simulink model "A2Model"  (R2015b)
settings: Solver=VariableStepAuto  StartTime=0.0  StopTime=inf  RelTol=1e-3
model workspace (MAT data in the model file):
  GPSLL = Simulink.Parameter
  GPSLL.Value = [47.255 11.345]
  GPSLL.DataType = 'auto'
  GPSLL.Units = 'auto'
  Inertia = Simulink.Parameter
  Inertia.Value = [0.035  0  0; 0  0.035  0; 0  0  0.011]
  Inertia.DataType = 'auto'
  Inertia.Units = 'auto'
  Mass = Simulink.Parameter
  Mass.Value = 1.5
  Mass.DataType = 'auto'
  Mass.Units = 'auto'
undefined symbols (not defined in the file): Earth, FilterK, PitchKd, PitchKi, PitchKp, PitchMax, Receive, RollKd, RollKi, RollKp, RollMax, Send, sigbuilder_block, Ts, WGS84
libraries: simulink x15, aerolibfltsims x5, simulink_extras x4, aerolibanimutils x2, aerolibtransform2 x2, aerolibconvert2 x2, aerolib6dof2 x1, aerolibatmos2 x1
settings Model: Creator=Ivan  LastModifiedBy=Ivan
settings OptimizationCC: DefaultParameterBehavior=Inlined  UseFloatMulNetSlope=on  InlineInvariantSignals=on  PassReuseOutputArgsAs=Individual arguments  ZeroExternalMemoryAtStartup=off  ZeroInternalMemoryAtStartup=off  NoFixptDivByZeroProtection=on  EfficientFloat2IntCast=on  OptimizeModelRefInitCode=on  LifeSpan=1
settings DebuggingCC: ParameterPrecisionLossMsg=none
settings HardwareCC: ProdBitPerPointer=32  ProdLargestAtomicInteger=Long  ProdLargestAtomicFloat=Double  ProdWordSize=32  ProdHWDeviceType=ARM Compatible->ARM Cortex
settings RTWCC: SystemTargetFile=ert.tlc  TemplateMakefile=ert_default_tmf  Description=Embedded Coder  GenerateReport=on  IncludeHyperlinkInReport=on  LaunchReport=on  TargetLang=C++  GenerateTraceInfo=on  GenerateTraceReport=on  GenerateTraceReportSl=on  GenerateTraceReportSf=on  GenerateTraceReportEml=on
settings CodeAppCC: ForceParamTrailComments=on  IgnoreCustomStorageClasses=off  SimulinkDataObjDesc=on  CustomSymbolStrGlobalVar=rt$N$M  CustomSymbolStrType=$N$M  CustomSymbolStrFcn=$N$M$F  CustomSymbolStrMacro=$N$M  InsertBlockDesc=on
settings ERTTargetCC: GenerateSampleERTMain=on  IncludeMdlTerminateFcn=off  CombineSignalStateStructs=on  MultiInstanceERTCode=on  CodeInterfacePackaging=C++ class  SupportNonFinite=off  SupportComplex=off  InlinedParameterPlacement=NonHierarchical  RootIOFormat=Structure reference  ERTCustomFileTemplate=example_file_process.tlc  ERTFilePackagingFormat=CompactWithDataFile

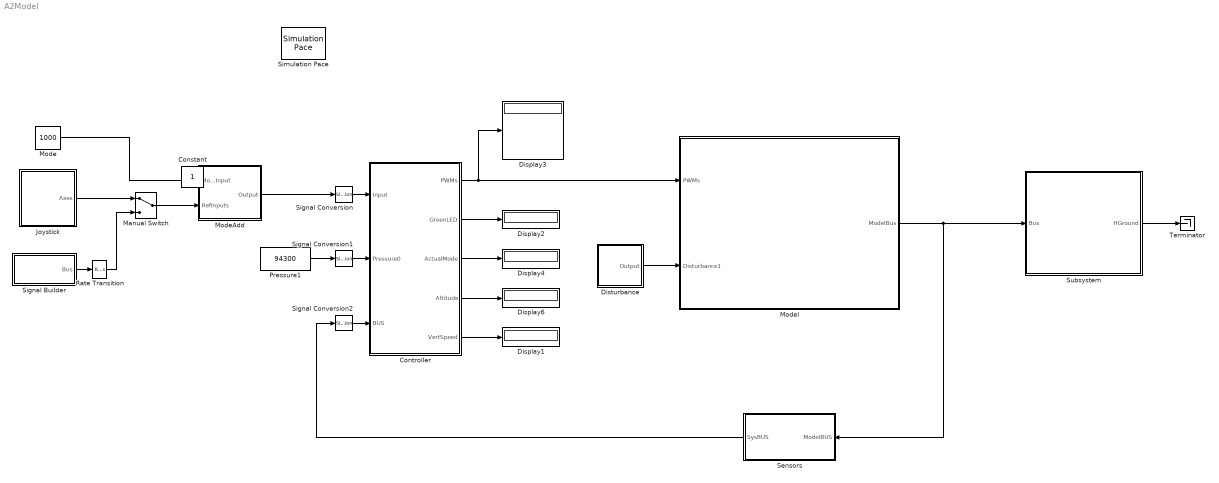
== system A2Model ==
  Controller : Subsystem  TreatAsAtomicUnit=on  SystemSampleTime=Ts
  Display{1..4,6} (5 alike) : Display
  Disturbance : Subsystem
  Joystick : Subsystem
  Manual Switch : ManualSwitch
  Mode : Constant  Value=1000  OutDataTypeStr=uint32  SampleTime=Ts
  ModeAdd : Subsystem
  Model : Subsystem
  Pressure1 : Constant  Value=94300  OutDataTypeStr=single  SampleTime=Ts
  Rate Transition : RateTransition  OutPortSampleTime=Ts
  Sensors : Subsystem
  Signal Conversion : SignalConversion
  Signal Conversion1 : SignalConversion
  Signal Conversion2 : SignalConversion
  Signal Builder : Subsystem  Tag=STV Subsys  LoadFcn=sigbuilder_block('load');  StartFcn=sigbuilder_block('start');  StopFcn=sigbuilder_block('stop');  ClipboardFcn=sigbuilder_block('clipboard');  mask(Sigbuilder block){}
      mask help: Simulink:masks:SigbuilderBlock_MD
      mask init:
      | if ~strcmp(get_param(bdroot(gcbh),'SimulationStatus'),'stopped') tuvar = sigbuilder_block('maskInit'); end
      settings: CopyFcn=sigbuilder_block('copy');  DeleteFcn=sigbuilder_block('delete');  ModelCloseFcn=sigbuilder_block('modelClose');  PreSaveFcn=sigbuilder_block('preSave');  PauseFcn=sigbuilder_block('pause');  ContinueFcn=sigbuilder_block('continue');  NameChangeFcn=sigbuilder_block('namechange');  OpenFcn=sigbuilder_block('open',[489.5 178 830 726.5 ]);  CloseFcn=sigbuilder_block('close');
      mask Display: plot(0, 0, 100, 100,[2, 2, 32, 32, 2], [68, 8, 8, 68, 68],[32, 2], [38, 38], [32, 19, 2],[53, 60, 44], [32, 17, 17, 2],[16, 16, 31, 31]);txt = getActiveGroup(gcbh);text(2, 100, txt,'verticalAlignment', 'top');
  Simulation Pace : aerolibanimutils/Simulation Pace  SimulationPace=1  SleepMode=MATLAB Thread  OutputPaceError=off  SampleTime=Ts
  Subsystem : Subsystem
  Terminator : Terminator
  Constant : Constant  IOType=siggen
  wires:
  Mode/1 -> ModeAdd/1(ModeInput)
  Joystick/1(Axes) -> Manual Switch/1
  Manual Switch/1 -> ModeAdd/2(RefInputs)
  Signal Builder/1(Bus) -> Rate Transition/1
  Rate Transition/1 -> Manual Switch/2
  Disturbance/1(Output) -> Model/2(Disturbance1)
  Controller/1(PWMs) -> Model/1(PWMs), Display3/1
  Model/1(ModelBus) -> Subsystem/1(Bus), Sensors/1(ModelBUS)
  Sensors/1(SysBUS) -> Signal Conversion2/1
  Controller/4(Altitude) -> Display6/1
  Controller/5(VertSpeed) -> Display1/1
  Controller/2(GreenLED) -> Display2/1
  Pressure1/1 -> Signal Conversion1/1
  Controller/3(ActualMode) -> Display4/1
  Signal Conversion/1 -> Controller/1(Input)
  Signal Conversion1/1 -> Controller/2(Pressure0)
  Signal Conversion2/1 -> Controller/3(BUS)
  Subsystem/1(HGround) -> Terminator/1
  ModeAdd/1(Output) -> Signal Conversion/1

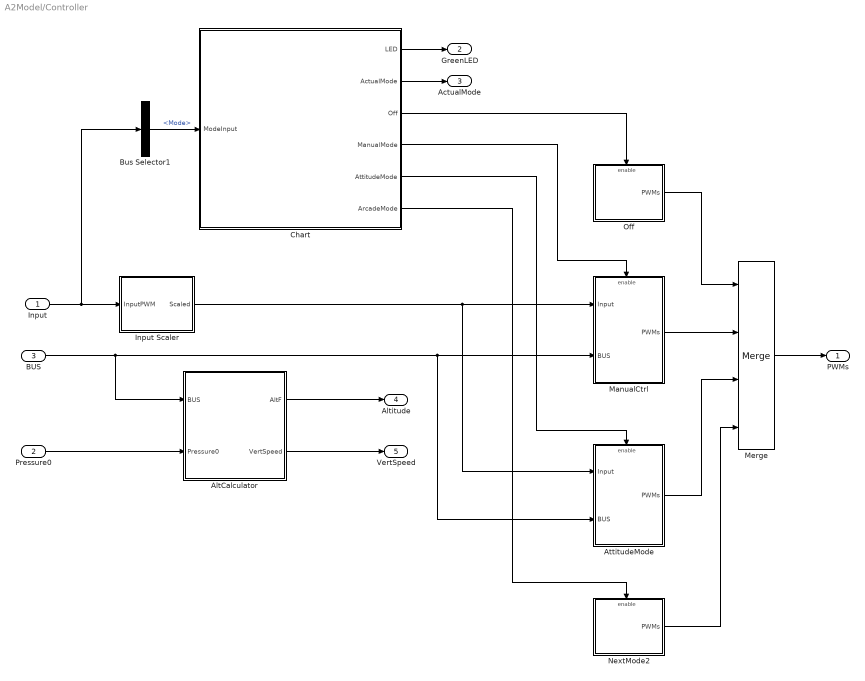
== system A2Model/Controller ==
  Input : Inport
  Pressure0 : Inport  Port=2
  BUS : Inport  Port=3
  AltCalculator : Subsystem
  AttitudeMode : Subsystem
  Bus Selector1 : BusSelector  OutputSignals=Mode
  Chart : Stateflow chart  TreatAsAtomicUnit=on
  Input Scaler : Subsystem
  ManualCtrl : Subsystem
  Merge : Merge  Inputs=4
  NextMode2 : Subsystem
  Off : Subsystem
  PWMs : Outport
  GreenLED : Outport  Port=2
  ActualMode : Outport  Port=3
  Altitude : Outport  Port=4
  VertSpeed : Outport  Port=5
  wires:
  Input/1 -> Bus Selector1/1, Input Scaler/1(InputPWM)
  BUS/1 -> ManualCtrl/2(BUS), AttitudeMode/2(BUS), AltCalculator/1(BUS)
  AltCalculator/2(VertSpeed) -> VertSpeed/1
  AltCalculator/1(AltF) -> Altitude/1
  Pressure0/1 -> AltCalculator/2(Pressure0)
  Input Scaler/1(Scaled) -> AttitudeMode/1(Input), ManualCtrl/1(Input)
  Chart/1(LED) -> GreenLED/1
  Bus Selector1/1 -> Chart/1(ModeInput)  "<Mode>"
  ManualCtrl/1(PWMs) -> Merge/2
  Off/1(PWMs) -> Merge/1
  Merge/1 -> PWMs/1
  Chart/2(ActualMode) -> ActualMode/1
  Chart/4(" ManualMode") -> ManualCtrl/Enable
  AttitudeMode/1(PWMs) -> Merge/3
  Chart/3(" Off") -> Off/Enable
  Chart/5(" AttitudeMode") -> AttitudeMode/Enable
  Chart/6(" ArcadeMode") -> NextMode2/Enable
  NextMode2/1(PWMs) -> Merge/4

== system A2Model/Disturbance ==
  Mode3 : Constant  Value=[0 0 0]  OutDataTypeStr=Inherit: Inherit via back propagation  SampleTime=Ts
  Mux : Mux  Inputs=2
  Step : Step  Time=10  Before=[0 0 0]  After=[0 0 0]  SampleTime=0
  Output : Outport
  wires:
  Step/1 -> Mux/1  "F[N]"
  Mux/1 -> Output/1
  Mode3/1 -> Mux/2  "Torque"

== system A2Model/Joystick ==
  Bus Creator : BusCreator  Inputs=4
  Joy Scaler : Subsystem
  Joystick : Subsystem
  Terminator{,1..3} (4 alike) : Terminator
  Axes : Outport
  wires:
  Joystick/1(Roll) -> Bus Creator/1  "Roll"
  Joystick/2(Pitch) -> Bus Creator/2  "Pitch"
  Joystick/3(Yaw) -> Bus Creator/3  "Yaw"
  Joystick/4(Throttle) -> Bus Creator/4  "Throttle"
  Bus Creator/1 -> Joy Scaler/1(Joystick)
  Joystick/7(B3) -> Terminator3/1
  Joystick/6(B2) -> Terminator1/1
  Joystick/5(B1) -> Terminator/1
  Joystick/8(B4) -> Terminator2/1
  Joy Scaler/1(Scaled) -> Axes/1

== system A2Model/ModeAdd ==
  ModeInput : Inport
  RefInputs : Inport  Port=2
  Bus Creator : BusCreator  Inputs=5
  Bus Selector2 : BusSelector  OutputSignals=Thr,Aileron,Elevator,Rudder
  Data Type Conversion{,1..3} (4 alike) : DataTypeConversion  OutDataTypeStr=single
  Output : Outport
  wires:
  Bus Selector2/1 -> Data Type Conversion/1  "<Thr>"
  Bus Selector2/2 -> Data Type Conversion1/1  "<Aileron>"
  RefInputs/1 -> Bus Selector2/1
  Bus Selector2/3 -> Data Type Conversion2/1  "<Elevator>"
  Bus Selector2/4 -> Data Type Conversion3/1  "<Rudder>"
  Bus Creator/1 -> Output/1
  ModeInput/1 -> Bus Creator/1  "Mode"
  Data Type Conversion/1 -> Bus Creator/2  "Thr"
  Data Type Conversion1/1 -> Bus Creator/3  "Aileron"
  Data Type Conversion2/1 -> Bus Creator/4  "Elevator"
  Data Type Conversion3/1 -> Bus Creator/5  "Rudder"

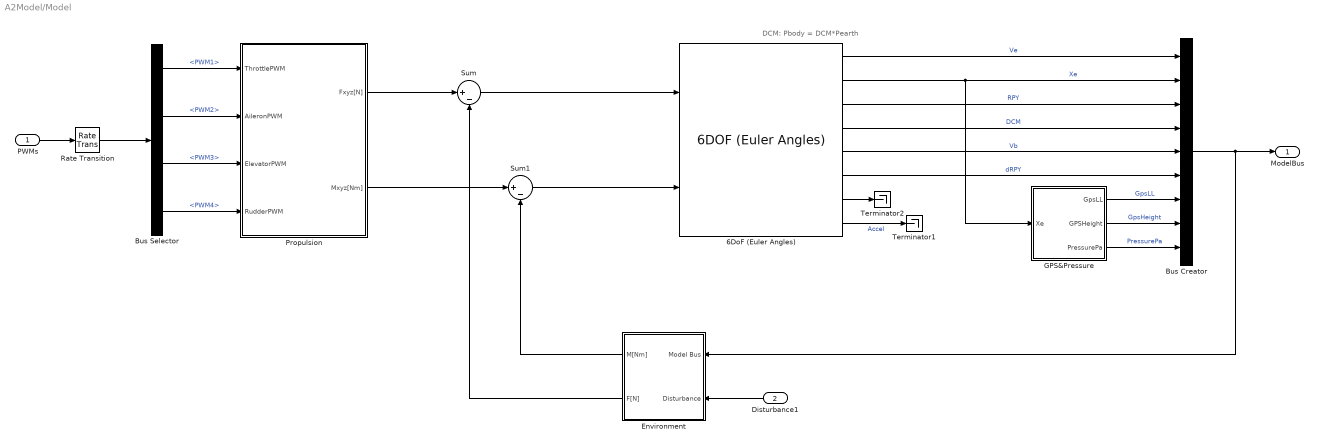
== system A2Model/Model ==
  note: DCM:
      | Pbody = DCM*Pearth
  PWMs : Inport
  Disturbance1 : Inport  Port=2
  6DoF (Euler Angles) : aerolib6dof2/6DOF (Euler Angles)  units=Metric (MKS)  mtype=Fixed  rep=Euler Angles  xme_0=[0 0 -600]  Vm_0=[0 0 0]  eul_0=[0 0 0]  pm_0=[0 0 0]  mass_0=Mass  mass_e=0.5  mass_f=2.0  inertia=Inertia  inertia_e=eye(3)  inertia_f=2*eye(3)  k_quat=1.0  vre_flag=on
  Bus Creator : BusCreator  Inputs=9
  Bus Selector : BusSelector  OutputSignals=PWM1,PWM2,PWM3,PWM4
  Environment : Subsystem
  GPS&Pressure : Subsystem
  Propulsion : Subsystem
  Rate Transition : RateTransition
  Sum : Sum  Inputs=|+-
  Sum1 : Sum  Inputs=|+-
  Terminator1 : Terminator
  Terminator2 : Terminator
  ModelBus : Outport
  wires:
  6DoF (Euler Angles)/1 -> Bus Creator/1  "Ve"
  6DoF (Euler Angles)/2 -> GPS&Pressure/1(Xe), Bus Creator/2  "Xe"
  6DoF (Euler Angles)/3 -> Bus Creator/3  "RPY"
  6DoF (Euler Angles)/4 -> Bus Creator/4  "DCM"
  Propulsion/2(Mxyz[Nm]) -> Sum1/1
  Propulsion/1(Fxyz[N]) -> Sum/1
  6DoF (Euler Angles)/7 -> Terminator2/1
  PWMs/1 -> Rate Transition/1
  Bus Selector/1 -> Propulsion/1(ThrottlePWM)  "<PWM1>"
  Bus Selector/2 -> Propulsion/2(AileronPWM)  "<PWM2>"
  Bus Selector/3 -> Propulsion/3(ElevatorPWM)  "<PWM3>"
  Bus Selector/4 -> Propulsion/4(RudderPWM)  "<PWM4>"
  Sum/1 -> 6DoF (Euler Angles)/1
  6DoF (Euler Angles)/5 -> Bus Creator/5  "Vb"
  6DoF (Euler Angles)/6 -> Bus Creator/6  "dRPY"
  Rate Transition/1 -> Bus Selector/1
  6DoF (Euler Angles)/8 -> Terminator1/1  "Accel"
  GPS&Pressure/1(GpsLL) -> Bus Creator/7  "GpsLL"
  GPS&Pressure/2(GPSHeight) -> Bus Creator/8  "GpsHeight"
  GPS&Pressure/3(PressurePa) -> Bus Creator/9  "PressurePa"
  Bus Creator/1 -> Environment/1(Model Bus), ModelBus/1
  Disturbance1/1 -> Environment/2(Disturbance)
  Sum1/1 -> 6DoF (Euler Angles)/2
  Environment/1(M[Nm]) -> Sum1/2
  Environment/2(F[N]) -> Sum/2

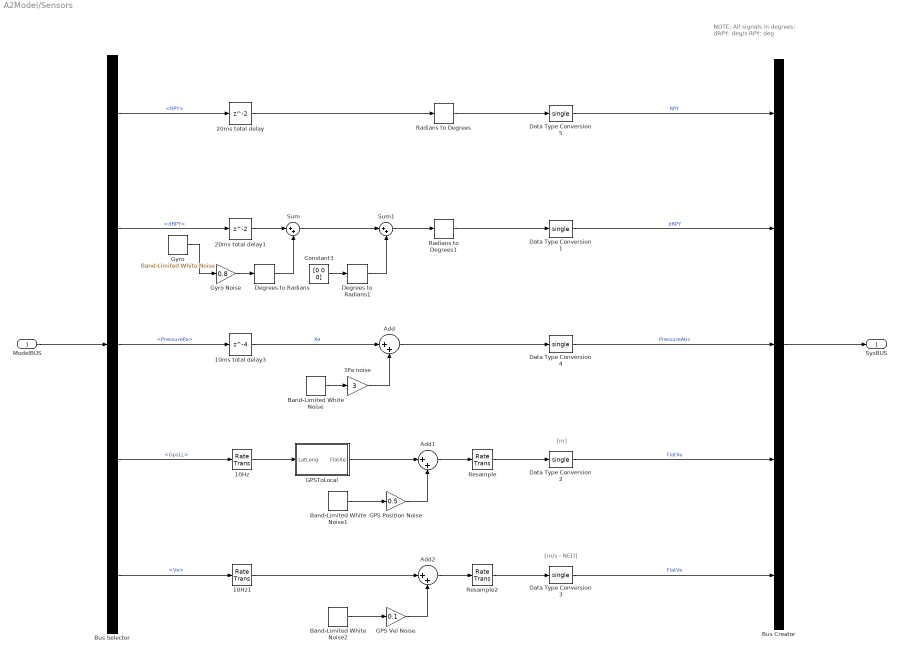
== system A2Model/Sensors ==
  note: [m/s - NED]
  note: [m]
  note: NOTE: All signals in degrees:
      | dRPY: deg/s
      | RPY: deg
  ModelBUS : Inport
  10Hz : RateTransition  OutPortSampleTime=1/10
  10Hz1 : RateTransition  OutPortSampleTime=1/10
  10ms total delay3 : Delay  DelayLength=4  SampleTime=Ts
  20ms total delay : Delay  SampleTime=Ts
  20ms total delay1 : Delay  SampleTime=Ts
  3Pa noise : Gain  Gain=3
  Add : Sum  Inputs=|++
  Add1 : Sum  Inputs=|++
  Add2 : Sum  Inputs=|++
  Band-Limited White Noise : simulink/Sources/Band-Limited White Noise  Cov=[1]*Ts  Ts=Ts  seed=[23341]
  Band-Limited White Noise1 : simulink/Sources/Band-Limited White Noise  Cov=[1]*Ts  Ts=Ts  seed=[23341]
  Band-Limited White Noise2 : simulink/Sources/Band-Limited White Noise  Cov=[1]*Ts  Ts=Ts  seed=[23341]
  Bus Creator : BusCreator  Inputs=5
  Bus Selector : BusSelector  OutputSignals=RPY,dRPY,PressurePa,GpsLL,Ve
  Constant3 : Constant  Value=[0 0 0]  OutDataTypeStr=single
  Data Type Conversion{1..5} (5 alike) : DataTypeConversion  OutDataTypeStr=single
  Degrees to Radians : simulink_extras/Transformations/Degrees to Radians
  Degrees to Radians1 : simulink_extras/Transformations/Degrees to Radians
  GPS Position Noise : Gain  Gain=0.5
  GPS Vel Noise : Gain  Gain=0.1
  GPSToLocal : Subsystem
  Gyro : simulink/Sources/Band-Limited White Noise  Cov=[1]*Ts  Ts=Ts  seed=[23341]
  Gyro Noise : Gain  Gain=0.8
  Radians to Degrees : simulink_extras/Transformations/Radians to Degrees
  Radians to Degrees1 : simulink_extras/Transformations/Radians to Degrees
  Resample : RateTransition  OutPortSampleTime=Ts
  Resample2 : RateTransition  OutPortSampleTime=Ts
  Sum : Sum  Inputs=|++
  Sum1 : Sum  Inputs=|++
  SysBUS : Outport
  wires:
  ModelBUS/1 -> Bus Selector/1
  Bus Selector/1 -> 20ms total delay/1  "<RPY>"
  Bus Creator/1 -> SysBUS/1
  Bus Selector/2 -> 20ms total delay1/1  "<dRPY>"
  20ms total delay/1 -> Radians to Degrees/1
  20ms total delay1/1 -> Sum/1
  Gyro/1 -> Gyro Noise/1
  Data Type Conversion5/1 -> Bus Creator/1  "RPY"
  Data Type Conversion1/1 -> Bus Creator/2  "dRPY"
  Degrees to Radians/1 -> Sum/2
  Radians to Degrees/1 -> Data Type Conversion5/1
  Radians to Degrees1/1 -> Data Type Conversion1/1
  Sum/1 -> Sum1/1
  Sum1/1 -> Radians to Degrees1/1
  Constant3/1 -> Degrees to Radians1/1
  Degrees to Radians1/1 -> Sum1/2
  Data Type Conversion3/1 -> Bus Creator/5  "FlatVe"
  Data Type Conversion2/1 -> Bus Creator/4  "FlatXe"
  3Pa noise/1 -> Add/2
  Band-Limited White Noise/1 -> 3Pa noise/1
  Add/1 -> Data Type Conversion4/1
  10ms total delay3/1 -> Add/1  "Xe"
  Bus Selector/3 -> 10ms total delay3/1  "<PressurePa>"
  Data Type Conversion4/1 -> Bus Creator/3  "PressureAbs"
  Bus Selector/4 -> 10Hz/1  "<GpsLL>"
  Bus Selector/5 -> 10Hz1/1  "<Ve>"
  10Hz/1 -> GPSToLocal/1(LatLong)
  Resample/1 -> Data Type Conversion2/1
  Resample2/1 -> Data Type Conversion3/1
  GPS Position Noise/1 -> Add1/2
  Band-Limited White Noise1/1 -> GPS Position Noise/1
  GPSToLocal/1(FlatXe) -> Add1/1
  Add1/1 -> Resample/1
  GPS Vel Noise/1 -> Add2/2
  Band-Limited White Noise2/1 -> GPS Vel Noise/1
  10Hz1/1 -> Add2/1
  Add2/1 -> Resample2/1
  Gyro Noise/1 -> Degrees to Radians/1

== system A2Model/Signal Builder ==
  Bus Creator : BusCreator  Tag=Bus Creator  Inputs=4
  FromWs : FromWorkspace  Tag=STV FromWs  VariableName=tuvar  SampleTime=0
      SigBuilderData=|
      | common.afterFinalStr = 'Extrapolate'
      | common.sampleTime = 0
      | dataSet.timeRange = [0 20]
      | dataSet.name = 'Group 1'
      | sbobj.Groups.Name = 'Group 1'
      | sbobj.Groups.Signals(1).Name = 'Thr'
      | sbobj.Groups.Signals(1).XData = [0 20]
      | sbobj.Groups.Signals(1).YData = [1300 1300]
      | sbobj.Groups.Signals(2).Name = 'Aileron'
      | sbobj.Groups.Signals(2).XData = [0 20]
      | sbobj.Groups.Signals(2).YData = [1024 1024]
      | sbobj.Groups.Signals(3).Name = 'Elevator'
      | sbobj.Groups.Signals(3).XData = [0 20]
      | sbobj.Groups.Signals(3).YData = [1024 1024]
      | sbobj.Groups.Signals(4).Name = 'Rudder'
      | sbobj.Groups.Signals(4).XData = [0 20]
      | sbobj.Groups.Signals(4).YData = [1024 1024]
      | sbobj.Groups.TimeRange = [0 20]
  Subsystem : Subsystem
  Bus : Outport
  wires:
  FromWs/1 -> Subsystem/1(In1)
  Subsystem/1(Thr) -> Bus Creator/1  "Thr"
  Subsystem/2(Aileron) -> Bus Creator/2  "Aileron"
  Subsystem/3(Elevator) -> Bus Creator/3  "Elevator"
  Subsystem/4(Rudder) -> Bus Creator/4  "Rudder"
  Bus Creator/1 -> Bus/1

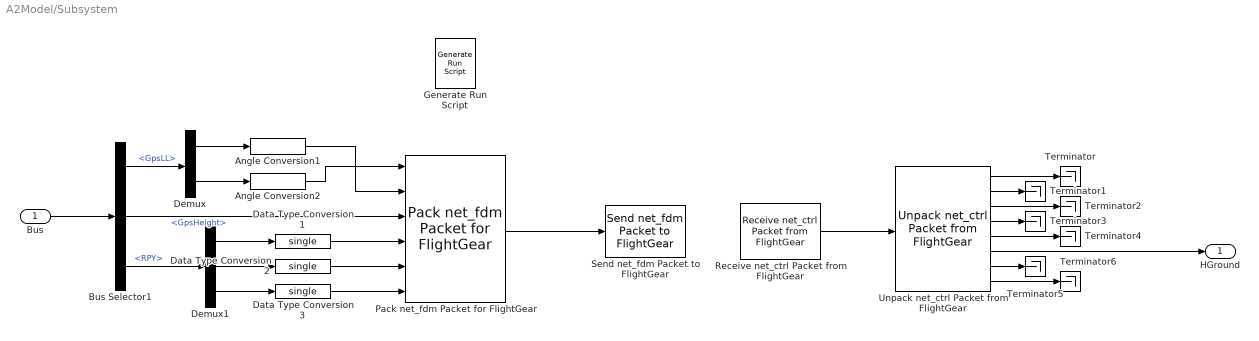
== system A2Model/Subsystem ==
  Bus : Inport
  Angle Conversion1 : aerolibconvert2/Angle Conversion  IU=deg  OU=rad
  Angle Conversion2 : aerolibconvert2/Angle Conversion  IU=deg  OU=rad
  Bus Selector1 : BusSelector  OutputSignals=GpsLL,GpsHeight,RPY
  Data Type Conversion1 : DataTypeConversion  OutDataTypeStr=single
  Data Type Conversion2 : DataTypeConversion  OutDataTypeStr=single
  Data Type Conversion3 : DataTypeConversion  OutDataTypeStr=single
  Demux : Demux  Outputs=2
  Demux1 : Demux  Outputs=3
  Generate Run Script : aerolibfltsims/Generate Run Script  OutputFileName=runfg.bat  FlightGearBaseDirectory=C:\Program Files\FlightGear 3.4.0  GeometryModelName=Kiki  DestinationPort=5502  OriginAddress=127.0.0.1  OriginPort=5505  LocalAddress=127.0.0.1  AirportId=LDZA  RunwayId=16  InitialAltitude=5000  InitialHeading=0  OffsetDistance=0  OffsetAzimuth=0  GenerateFile=off  Architecture=Win64  dataFlow=Send-Receive
  Pack net_fdm Packet for FlightGear : aerolibfltsims/Pack net_fdm Packet for FlightGear  FlightGearVersion=v3.4  ShowPositionAttitudeInputs=on  ShowVelocityAccelerationInputs=off  ShowControlSurfacePositionInputs=off  ShowEngineFuelInputs=off  ShowLandingGearInputs=off  ShowEnvironmentInputs=off  SampleTime=1/30
  Receive net_ctrl Packet from FlightGear : aerolibfltsims/Receive net_ctrl Packet from FlightGear  FlightGearVersion=v3.4  ReceiveAddress=127.0.0.1  ReceivePort=5505  ReceiveWidth=744  varLen=off  SampleTime=1/30  packetFlag=off
      settings: AttributesFormatString=Version Selected:\n%<FlightGearVersion>
  Send net_fdm Packet to FlightGear : aerolibfltsims/Send net_fdm Packet to FlightGear  DestinationIpAddress=127.0.0.1  DestinationPort=5502  LocalIpPort=-1  varLen=off  SampleTime=1/30
  Terminator{,1..6} (7 alike) : Terminator
  Unpack net_ctrl Packet from FlightGear : aerolibfltsims/Unpack net_ctrl Packet from FlightGear  FlightGearVersion=v3.4  ShowControlSurfacePositionOutputs=off  ShowEngineFuelOutputs=off  ShowLandingGearOutputs=off  ShowAvionicOutputs=off  ShowEnvironmentOutputs=on  SampleTime=1/30
      settings: AttributesFormatString=Version Selected: %<FlightGearVersion>
  HGround : Outport
  wires:
  Pack net_fdm Packet for FlightGear/1 -> Send net_fdm Packet to FlightGear/1
  Bus/1 -> Bus Selector1/1
  Bus Selector1/1 -> Demux/1  "<GpsLL>"
  Demux/1 -> Angle Conversion1/1
  Demux/2 -> Angle Conversion2/1
  Bus Selector1/2 -> Pack net_fdm Packet for FlightGear/3  "<GpsHeight>"
  Demux1/1 -> Data Type Conversion1/1
  Demux1/2 -> Data Type Conversion2/1
  Demux1/3 -> Data Type Conversion3/1
  Data Type Conversion1/1 -> Pack net_fdm Packet for FlightGear/4
  Data Type Conversion2/1 -> Pack net_fdm Packet for FlightGear/5
  Data Type Conversion3/1 -> Pack net_fdm Packet for FlightGear/6
  Bus Selector1/3 -> Demux1/1  "<RPY>"
  Receive net_ctrl Packet from FlightGear/1 -> Unpack net_ctrl Packet from FlightGear/1
  Unpack net_ctrl Packet from FlightGear/6 -> HGround/1
  Angle Conversion1/1 -> Pack net_fdm Packet for FlightGear/2
  Angle Conversion2/1 -> Pack net_fdm Packet for FlightGear/1
  Unpack net_ctrl Packet from FlightGear/1 -> Terminator/1
  Unpack net_ctrl Packet from FlightGear/2 -> Terminator1/1
  Unpack net_ctrl Packet from FlightGear/3 -> Terminator2/1
  Unpack net_ctrl Packet from FlightGear/4 -> Terminator3/1
  Unpack net_ctrl Packet from FlightGear/5 -> Terminator4/1
  Unpack net_ctrl Packet from FlightGear/7 -> Terminator5/1
  Unpack net_ctrl Packet from FlightGear/8 -> Terminator6/1

== system A2Model/Controller/AltCalculator ==
  BUS : Inport
  Pressure0 : Inport  Port=2
  Bus Selector1 : BusSelector  OutputSignals=PressureAbs
  Delay : Delay  DelayLength=100
  Discrete FIR Filter : DiscreteFir  Coefficients=FilterK
  Gain : Gain  Gain=1/(100*Ts)
  MATLAB Function : MATLAB Function  TreatAsAtomicUnit=on
  Sum : Sum  Inputs=|+-
  AltF : Outport
  VertSpeed : Outport  Port=2
  wires:
  BUS/1 -> Bus Selector1/1
  Bus Selector1/1 -> MATLAB Function/1(pressure)  "<PressureAbs>"
  MATLAB Function/1(alt) -> Discrete FIR Filter/1
  Sum/1 -> Gain/1
  Discrete FIR Filter/1 -> Delay/1, Sum/1, AltF/1
  Delay/1 -> Sum/2
  Gain/1 -> VertSpeed/1
  Pressure0/1 -> MATLAB Function/2(pressure0)

== system A2Model/Controller/AttitudeMode ==
  Input : Inport  OutDataTypeStr=single
  BUS : Inport  Port=2  OutDataTypeStr=single
  Enable : EnablePort  StatesWhenEnabling=reset
  Bus Selector1 : BusSelector  OutputSignals=Thr,Aileron,Elevator,Rudder
  Gain : Gain
  Gain3 : Gain
  Mapper : Subsystem
  PitchController : Subsystem
  RollController : Subsystem
  PWMs : Outport
  wires:
  Mapper/1(PwmOut) -> PWMs/1
  Gain/1 -> Mapper/1(Thr)
  Gain3/1 -> Mapper/4(Rudder)
  PitchController/1(PitchOut) -> Mapper/3(Elevator)
  Bus Selector1/4 -> Gain3/1  "<Rudder>"
  Input/1 -> Bus Selector1/1
  Bus Selector1/1 -> Gain/1  "<Thr>"
  Bus Selector1/3 -> PitchController/2(PitchRef)  "<Elevator>"
  BUS/1 -> PitchController/1(Bus), RollController/1(Bus)
  Bus Selector1/2 -> RollController/2(RollRef)  "<Aileron>"
  RollController/1(RollOut) -> Mapper/2(Aileron)

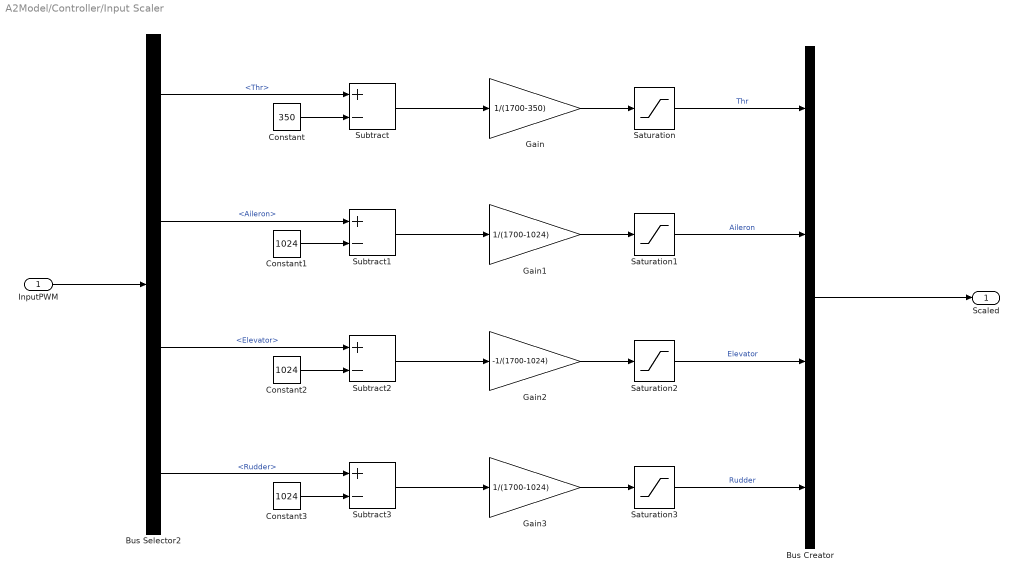
== system A2Model/Controller/Input Scaler ==
  InputPWM : Inport
  Bus Creator : BusCreator  Inputs=4
  Bus Selector2 : BusSelector  OutputSignals=Thr,Aileron,Elevator,Rudder
  Constant : Constant  Value=350  OutDataTypeStr=single
  Constant1 : Constant  Value=1024  OutDataTypeStr=single
  Constant2 : Constant  Value=1024  OutDataTypeStr=single
  Constant3 : Constant  Value=1024  OutDataTypeStr=single
  Gain : Gain  Gain=1/(1700-350)
  Gain1 : Gain  Gain=1/(1700-1024)
  Gain2 : Gain  Gain=-1/(1700-1024)
  Gain3 : Gain  Gain=1/(1700-1024)
  Saturation : Saturate  UpperLimit=1  LowerLimit=0
  Saturation1 : Saturate  UpperLimit=1  LowerLimit=-1
  Saturation2 : Saturate  UpperLimit=1  LowerLimit=-1
  Saturation3 : Saturate  UpperLimit=1  LowerLimit=-1
  Subtract{,1..3} (4 alike) : Sum  Inputs=+-
  Scaled : Outport
  wires:
  Bus Creator/1 -> Scaled/1
  InputPWM/1 -> Bus Selector2/1
  Bus Selector2/1 -> Subtract/1  "<Thr>"
  Constant/1 -> Subtract/2
  Subtract/1 -> Gain/1
  Gain/1 -> Saturation/1
  Saturation/1 -> Bus Creator/1  "Thr"
  Bus Selector2/2 -> Subtract1/1  "<Aileron>"
  Constant1/1 -> Subtract1/2
  Subtract1/1 -> Gain1/1
  Gain1/1 -> Saturation1/1
  Saturation1/1 -> Bus Creator/2  "Aileron"
  Bus Selector2/3 -> Subtract2/1  "<Elevator>"
  Constant2/1 -> Subtract2/2
  Subtract2/1 -> Gain2/1
  Gain2/1 -> Saturation2/1
  Saturation2/1 -> Bus Creator/3  "Elevator"
  Bus Selector2/4 -> Subtract3/1  "<Rudder>"
  Constant3/1 -> Subtract3/2
  Subtract3/1 -> Gain3/1
  Gain3/1 -> Saturation3/1
  Saturation3/1 -> Bus Creator/4  "Rudder"

== system A2Model/Controller/ManualCtrl ==
  Input : Inport  OutDataTypeStr=single
  BUS : Inport  Port=2  OutDataTypeStr=single
  Enable : EnablePort  StatesWhenEnabling=reset
  Bus Selector1 : BusSelector  OutputSignals=Thr,Aileron,Elevator,Rudder
  Gain{,1..3} (4 alike) : Gain
  Mapper : Subsystem
  Terminator : Terminator
  PWMs : Outport
  wires:
  Bus Selector1/4 -> Gain3/1  "<Rudder>"
  Input/1 -> Bus Selector1/1
  Bus Selector1/1 -> Gain/1  "<Thr>"
  Bus Selector1/3 -> Gain2/1  "<Elevator>"
  Bus Selector1/2 -> Gain1/1  "<Aileron>"
  BUS/1 -> Terminator/1
  Gain/1 -> Mapper/1(Thr)
  Gain1/1 -> Mapper/2(Aileron)
  Gain2/1 -> Mapper/3(Elevator)
  Gain3/1 -> Mapper/4(Rudder)
  Mapper/1(PwmOut) -> PWMs/1

== system A2Model/Controller/NextMode2 ==
  Enable : EnablePort  StatesWhenEnabling=reset
  Constant : Constant  Value=0.02  OutDataTypeStr=single
  Constant1 : Constant  Value=0  OutDataTypeStr=single
  Constant2 : Constant  Value=0  OutDataTypeStr=single
  Constant3 : Constant  Value=0  OutDataTypeStr=single
  Mapper : Subsystem
  PWMs : Outport
  wires:
  Mapper/1(PwmOut) -> PWMs/1
  Constant/1 -> Mapper/1(Thr)
  Constant3/1 -> Mapper/4(Rudder)
  Constant2/1 -> Mapper/3(Elevator)
  Constant1/1 -> Mapper/2(Aileron)

== system A2Model/Controller/Off ==
  Enable : EnablePort  StatesWhenEnabling=reset
  Constant{,1..3} (4 alike) : Constant  Value=0  OutDataTypeStr=single
  Mapper : Subsystem
  PWMs : Outport
  wires:
  Mapper/1(PwmOut) -> PWMs/1
  Constant/1 -> Mapper/1(Thr)
  Constant3/1 -> Mapper/4(Rudder)
  Constant2/1 -> Mapper/3(Elevator)
  Constant1/1 -> Mapper/2(Aileron)

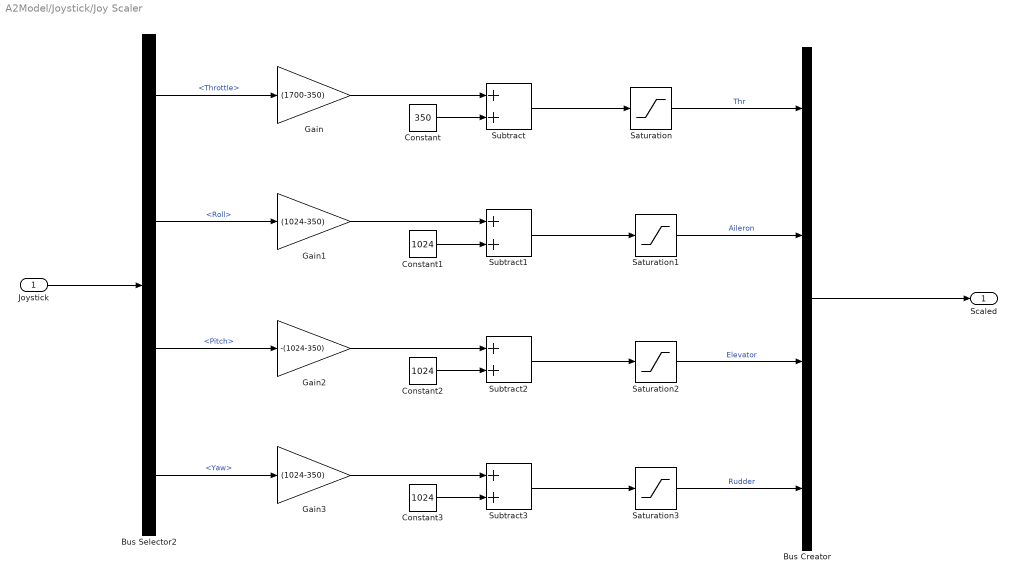
== system A2Model/Joystick/Joy Scaler ==
  Joystick : Inport
  Bus Creator : BusCreator  Inputs=4
  Bus Selector2 : BusSelector  OutputSignals=Throttle,Roll,Pitch,Yaw
  Constant : Constant  Value=350  OutDataTypeStr=single
  Constant1 : Constant  Value=1024  OutDataTypeStr=single
  Constant2 : Constant  Value=1024  OutDataTypeStr=single
  Constant3 : Constant  Value=1024  OutDataTypeStr=single
  Gain : Gain  Gain=(1700-350)
  Gain1 : Gain  Gain=(1024-350)
  Gain2 : Gain  Gain=-(1024-350)
  Gain3 : Gain  Gain=(1024-350)
  Saturation{,1..3} (4 alike) : Saturate  UpperLimit=1700  LowerLimit=350  OutDataTypeStr=Inherit: Inherit via back propagation
  Subtract{,1..3} (4 alike) : Sum
  Scaled : Outport
  wires:
  Bus Creator/1 -> Scaled/1
  Joystick/1 -> Bus Selector2/1
  Bus Selector2/1 -> Gain/1  "<Throttle>"
  Constant/1 -> Subtract/2
  Saturation/1 -> Bus Creator/1  "Thr"
  Gain/1 -> Subtract/1
  Subtract/1 -> Saturation/1
  Constant1/1 -> Subtract1/2
  Saturation1/1 -> Bus Creator/2  "Aileron"
  Gain1/1 -> Subtract1/1
  Subtract1/1 -> Saturation1/1
  Bus Selector2/2 -> Gain1/1  "<Roll>"
  Constant2/1 -> Subtract2/2
  Saturation2/1 -> Bus Creator/3  "Elevator"
  Gain2/1 -> Subtract2/1
  Subtract2/1 -> Saturation2/1
  Bus Selector2/3 -> Gain2/1  "<Pitch>"
  Constant3/1 -> Subtract3/2
  Saturation3/1 -> Bus Creator/4  "Rudder"
  Gain3/1 -> Subtract3/1
  Subtract3/1 -> Saturation3/1
  Bus Selector2/4 -> Gain3/1  "<Yaw>"

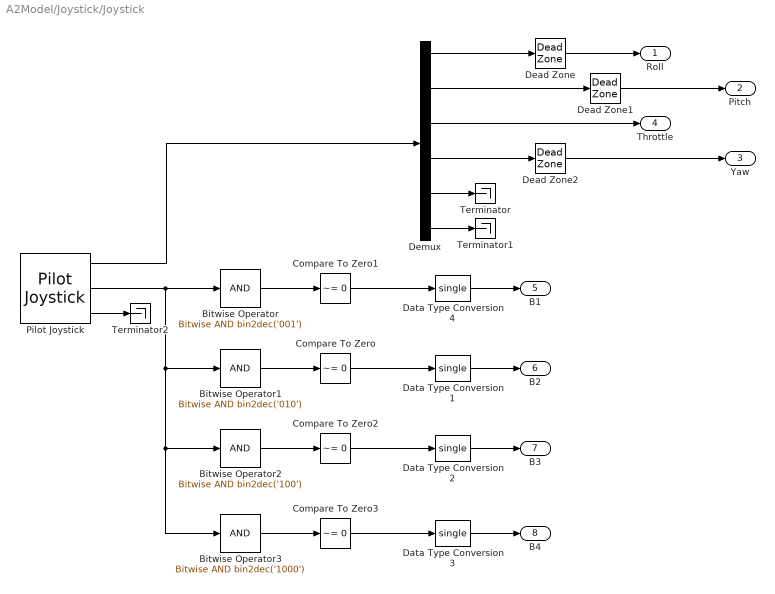
== system A2Model/Joystick/Joystick ==
  Bitwise Operator : simulink/Logic and Bit Operations/Bitwise Operator  logicop=AND  UseBitMask=on  BitMask=bin2dec('001')  BitMaskRealWorld=Stored Integer
  Bitwise Operator1 : simulink/Logic and Bit Operations/Bitwise Operator  logicop=AND  UseBitMask=on  BitMask=bin2dec('010')  BitMaskRealWorld=Stored Integer
  Bitwise Operator2 : simulink/Logic and Bit Operations/Bitwise Operator  logicop=AND  UseBitMask=on  BitMask=bin2dec('100')  BitMaskRealWorld=Stored Integer
  Bitwise Operator3 : simulink/Logic and Bit Operations/Bitwise Operator  logicop=AND  UseBitMask=on  BitMask=bin2dec('1000')  BitMaskRealWorld=Stored Integer
  Compare To Zero{,1..3} (4 alike) : simulink/Logic and Bit Operations/Compare To Zero  relop=~=  OutDataTypeStr=uint8
  Data Type Conversion{1..4} (4 alike) : DataTypeConversion  OutDataTypeStr=single
  Dead Zone : DeadZone  LowerValue=-0.12  UpperValue=0.12  SaturateOnIntegerOverflow=on
  Dead Zone1 : DeadZone  LowerValue=-0.12  UpperValue=0.12  SaturateOnIntegerOverflow=on
  Dead Zone2 : DeadZone  LowerValue=-0.12  UpperValue=0.12  SaturateOnIntegerOverflow=on
  Demux : Demux  Outputs=6
  Pilot Joystick : aerolibanimutils/Pilot Joystick  JoystickID=None  OutputConfiguration=AllOutputs  SampleTime=Ts
  Terminator : Terminator
  Terminator1 : Terminator
  Terminator2 : Terminator
  Roll : Outport
  Pitch : Outport  Port=2
  Yaw : Outport  Port=3
  Throttle : Outport  Port=4
  B1 : Outport  Port=5
  B2 : Outport  Port=6
  B3 : Outport  Port=7
  B4 : Outport  Port=8
  wires:
  Pilot Joystick/2 -> Bitwise Operator/1, Bitwise Operator1/1, Bitwise Operator2/1, Bitwise Operator3/1
  Demux/1 -> Dead Zone/1
  Demux/2 -> Dead Zone1/1
  Demux/4 -> Dead Zone2/1
  Demux/3 -> Throttle/1
  Bitwise Operator/1 -> Compare To Zero1/1
  Bitwise Operator1/1 -> Compare To Zero/1
  Compare To Zero/1 -> Data Type Conversion1/1
  Bitwise Operator2/1 -> Compare To Zero2/1
  Compare To Zero2/1 -> Data Type Conversion2/1
  Bitwise Operator3/1 -> Compare To Zero3/1
  Compare To Zero3/1 -> Data Type Conversion3/1
  Data Type Conversion1/1 -> B2/1
  Data Type Conversion2/1 -> B3/1
  Data Type Conversion3/1 -> B4/1
  Compare To Zero1/1 -> Data Type Conversion4/1
  Data Type Conversion4/1 -> B1/1
  Pilot Joystick/1 -> Demux/1
  Demux/6 -> Terminator1/1
  Demux/5 -> Terminator/1
  Pilot Joystick/3 -> Terminator2/1
  Dead Zone/1 -> Roll/1
  Dead Zone1/1 -> Pitch/1
  Dead Zone2/1 -> Yaw/1

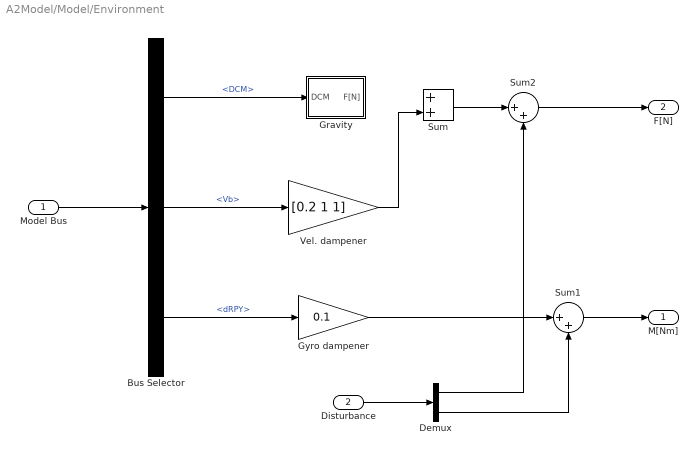
== system A2Model/Model/Environment ==
  Model Bus : Inport
  Disturbance : Inport  Port=2
  Bus Selector : BusSelector  OutputSignals=DCM,Vb,dRPY
  Demux : Demux  Outputs=2
  Gravity : Subsystem
  Gyro dampener : Gain  Gain=0.1
  Sum : Sum
  Sum1 : Sum  Inputs=|++
  Sum2 : Sum  Inputs=|++
  Vel. dampener : Gain  Gain=[0.2 1 1]
  M[Nm] : Outport
  F[N] : Outport  Port=2
  wires:
  Model Bus/1 -> Bus Selector/1
  Bus Selector/1 -> Gravity/1(DCM)  "<DCM>"
  Bus Selector/3 -> Gyro dampener/1  "<dRPY>"
  Bus Selector/2 -> Vel. dampener/1  "<Vb>"
  Vel. dampener/1 -> Sum/2
  Sum/1 -> Sum2/1
  Sum2/1 -> F[N]/1
  Gyro dampener/1 -> Sum1/1
  Sum1/1 -> M[Nm]/1
  Disturbance/1 -> Demux/1
  Demux/1 -> Sum2/2
  Demux/2 -> Sum1/2

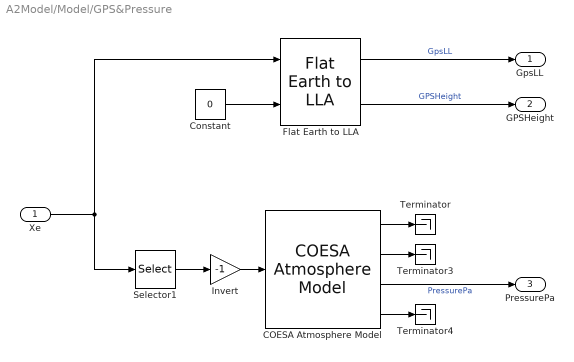
== system A2Model/Model/GPS&Pressure ==
  Xe : Inport
  COESA Atmosphere Model : aerolibatmos2/COESA Atmosphere Model  units=Metric (MKS)  spec=1976 COESA-extended U.S. Standard Atmosphere  model=Profile  profile_var=High temperature  profile_percent=1%  profile_alt=5 km (16404 ft)  envelope_var=High temperature  envelope_percent=1%  action=Warning
  Constant : Constant  Value=0
  Flat Earth to LLA : aerolibtransform2/Flat Earth to LLA  units=Metric (MKS)  ptype=Earth (WGS84)  F=1/298.257223563  R=6378137  LL0=GPSLL  psi=0
  Invert : Gain  Gain=-1
  Selector1 : Selector  InputPortWidth=3  IndexOptions=Index vector (dialog)  Indices=[3]  OutputSizes=1
  Terminator : Terminator
  Terminator3 : Terminator
  Terminator4 : Terminator
  GpsLL : Outport
  GPSHeight : Outport  Port=2
  PressurePa : Outport  Port=3
  wires:
  COESA Atmosphere Model/4 -> Terminator4/1
  COESA Atmosphere Model/2 -> Terminator3/1
  Xe/1 -> Flat Earth to LLA/1, Selector1/1
  Invert/1 -> COESA Atmosphere Model/1
  Selector1/1 -> Invert/1
  COESA Atmosphere Model/1 -> Terminator/1
  Flat Earth to LLA/1 -> GpsLL/1  "GpsLL"
  COESA Atmosphere Model/3 -> PressurePa/1  "PressurePa"
  Flat Earth to LLA/2 -> GPSHeight/1  "GPSHeight"
  Constant/1 -> Flat Earth to LLA/2

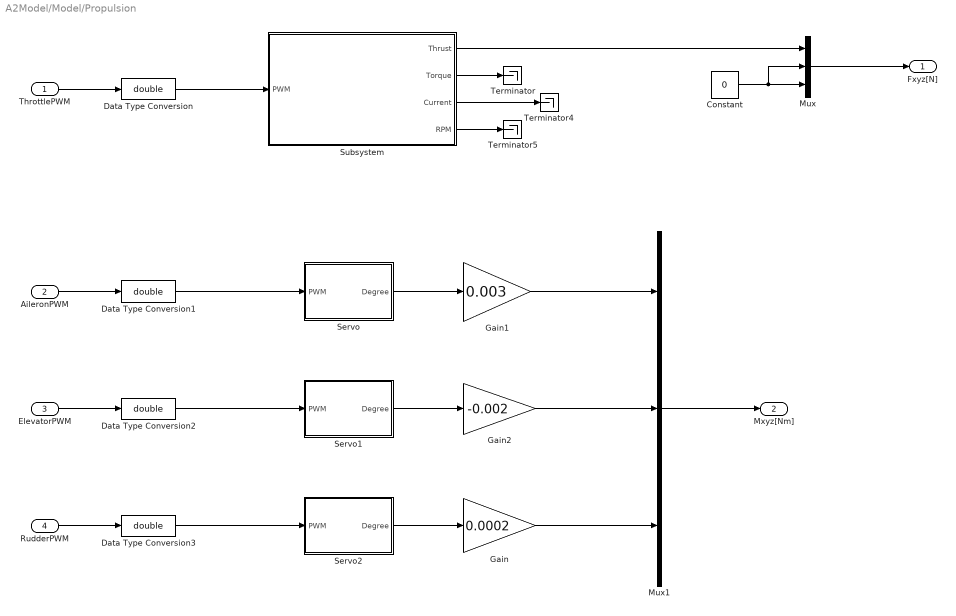
== system A2Model/Model/Propulsion ==
  ThrottlePWM : Inport
  AileronPWM : Inport  Port=2
  ElevatorPWM : Inport  Port=3
  RudderPWM : Inport  Port=4
  Constant : Constant  Value=0
  Data Type Conversion{,1..3} (4 alike) : DataTypeConversion  OutDataTypeStr=double
  Gain : Gain  Gain=0.0002
  Gain1 : Gain  Gain=0.003
  Gain2 : Gain  Gain=-0.002
  Mux : Mux  Inputs=3
  Mux1 : Mux  Inputs=3
  Servo : Subsystem
  Servo1 : Subsystem
  Servo2 : Subsystem
  Subsystem : Subsystem
  Terminator : Terminator
  Terminator4 : Terminator
  Terminator5 : Terminator
  Fxyz[N] : Outport
  Mxyz[Nm] : Outport  Port=2
  wires:
  ThrottlePWM/1 -> Data Type Conversion/1
  AileronPWM/1 -> Data Type Conversion1/1
  ElevatorPWM/1 -> Data Type Conversion2/1
  RudderPWM/1 -> Data Type Conversion3/1
  Mux/1 -> Fxyz[N]/1
  Subsystem/1(Thrust) -> Mux/1
  Constant/1 -> Mux/2, Mux/3
  Subsystem/2(Torque) -> Terminator/1
  Subsystem/3(Current) -> Terminator4/1
  Subsystem/4(RPM) -> Terminator5/1
  Servo/1(Degree) -> Gain1/1
  Data Type Conversion/1 -> Subsystem/1(PWM)
  Data Type Conversion1/1 -> Servo/1(PWM)
  Servo1/1(Degree) -> Gain2/1
  Data Type Conversion2/1 -> Servo1/1(PWM)
  Servo2/1(Degree) -> Gain/1
  Data Type Conversion3/1 -> Servo2/1(PWM)
  Mux1/1 -> Mxyz[Nm]/1
  Gain/1 -> Mux1/3
  Gain2/1 -> Mux1/2
  Gain1/1 -> Mux1/1

== system A2Model/Sensors/GPSToLocal ==
  LatLong : Inport
  Constant : Constant  Value=0
  LLA to Flat Earth : aerolibtransform2/LLA to Flat Earth  units=Metric (MKS)  ptype=Earth (WGS84)  F=1/298.257223563  R=6378137  LL0=GPSLL  psi=0
  Selector : Selector  InputPortWidth=3  IndexOptions=Index vector (dialog)  Indices=[1 2]  OutputSizes=1
  FlatXe : Outport
  wires:
  LatLong/1 -> LLA to Flat Earth/1
  Constant/1 -> LLA to Flat Earth/2, LLA to Flat Earth/3
  LLA to Flat Earth/1 -> Selector/1
  Selector/1 -> FlatXe/1

== system A2Model/Signal Builder/Subsystem ==
  In1 : Inport
  Demux : Demux  Tag=STV Demux
  Thr : Outport  Tag=STV Outport
  Aileron : Outport  Tag=STV Outport  Port=2
  Elevator : Outport  Tag=STV Outport  Port=3
  Rudder : Outport  Tag=STV Outport  Port=4
  wires:
  Demux/1 -> Thr/1
  Demux/2 -> Aileron/1
  Demux/3 -> Elevator/1
  Demux/4 -> Rudder/1
  In1/1 -> Demux/1

== system A2Model/Controller/AttitudeMode/Mapper ==
  Thr : Inport
  Aileron : Inport  Port=2
  Elevator : Inport  Port=3
  Rudder : Inport  Port=4
  Bus Creator1 : BusCreator  Inputs=4
  Gain2 : Gain  Gain=-1
  LimitAndRescale : Subsystem
  LimitAndRescale1 : Subsystem
  LimitAndRescale2 : Subsystem
  LimitAndRescale3 : Subsystem
  PwmOut : Outport
  wires:
  LimitAndRescale3/1(ESCPWM) -> Bus Creator1/4  "PWM4"
  LimitAndRescale2/1(ESCPWM) -> Bus Creator1/3  "PWM3"
  Bus Creator1/1 -> PwmOut/1
  LimitAndRescale/1(ESCPWM) -> Bus Creator1/1  "PWM1"
  LimitAndRescale1/1(ESCPWM) -> Bus Creator1/2  "PWM2"
  Thr/1 -> LimitAndRescale/1(Scaled)
  Elevator/1 -> Gain2/1
  Aileron/1 -> LimitAndRescale1/1(Scaled)
  Gain2/1 -> LimitAndRescale2/1(Scaled)
  Rudder/1 -> LimitAndRescale3/1(Scaled)

== system A2Model/Controller/AttitudeMode/PitchController ==
  Bus : Inport
  PitchRef : Inport  Port=2
  Bus Selector : BusSelector  OutputSignals=RPY
  Discrete PID Controller : simulink/Continuous/PID Controller  Controller=PID  TimeDomain=Discrete-time  SampleTime=Ts  IntegratorMethod=Forward Euler  FilterMethod=Forward Euler  Form=Parallel  UseFilter=on  ControllerParametersSource=internal  P=PitchKp  I=PitchKi  D=PitchKd  N=50  InitialConditionSource=internal  InitialConditionForIntegrator=0  InitialConditionForFilter=0  ExternalReset=none  LimitOutput=on  UpperSaturationLimit=1  LowerSaturationLimit=-1  LinearizeAsGain=off  AntiWindupMode=clamping  Kb=1  TrackingMode=off  Kt=1  PParamMin=[]  PParamMax=[]  IParamMin=[]  IParamMax=[]  DParamMin=[]  DParamMax=[]  NParamMin=[]  NParamMax=[]  KbParamMin=[]  KbParamMax=[]  KtParamMin=[]  KtParamMax=[]  POutMin=[]  POutMax=[]  IOutMin=[]  IOutMax=[]  DOutMin=[]  DOutMax=[]  NOutMin=[]  NOutMax=[]  KbOutMin=[]  KbOutMax=[]  KtOutMin=[]  KtOutMax=[]  IntegratorOutMin=[]  IntegratorOutMax=[]  FilterOutMin=[]  FilterOutMax=[]  SumOutMin=[]  SumOutMax=[]  SumI1OutMin=[]  SumI1OutMax=[]  SumI2OutMin=[]  SumI2OutMax=[]  SumI3OutMin=[]  SumI3OutMax=[]  SumDOutMin=[]  SumDOutMax=[]  SaturationOutMin=[]  SaturationOutMax=[]  IntegratorContinuousStateAttributes=''  IntegratorStateMustResolveToSignalObject=off  IntegratorRTWStateStorageClass=Auto  FilterContinuousStateAttributes=''  FilterStateMustResolveToSignalObject=off  FilterRTWStateStorageClass=Auto  DifferentiatorICPrevScaledInput=0  DifferentiatorOutMin=[]  DifferentiatorOutMax=[]
  Scale : Gain  Gain=PitchMax
  Selector3 : Selector  InputPortWidth=3  IndexOptions=Index vector (dialog)  Indices=[2]  OutputSizes=1
  Sum : Sum  Inputs=|+-
  PitchOut : Outport
  wires:
  Discrete PID Controller/1 -> PitchOut/1
  Bus Selector/1 -> Selector3/1  "<RPY>"
  Selector3/1 -> Sum/2
  PitchRef/1 -> Scale/1
  Bus/1 -> Bus Selector/1
  Scale/1 -> Sum/1
  Sum/1 -> Discrete PID Controller/1

== system A2Model/Controller/AttitudeMode/RollController ==
  Bus : Inport
  RollRef : Inport  Port=2
  Bus Selector : BusSelector  OutputSignals=RPY
  Discrete PID Controller : simulink/Continuous/PID Controller  Controller=PID  TimeDomain=Discrete-time  SampleTime=Ts  IntegratorMethod=Forward Euler  FilterMethod=Forward Euler  Form=Parallel  UseFilter=on  ControllerParametersSource=internal  P=RollKp  I=RollKi  D=RollKd  N=50  InitialConditionSource=internal  InitialConditionForIntegrator=0  InitialConditionForFilter=0  ExternalReset=none  LimitOutput=on  UpperSaturationLimit=1  LowerSaturationLimit=-1  LinearizeAsGain=off  AntiWindupMode=clamping  Kb=1  TrackingMode=off  Kt=1  PParamMin=[]  PParamMax=[]  IParamMin=[]  IParamMax=[]  DParamMin=[]  DParamMax=[]  NParamMin=[]  NParamMax=[]  KbParamMin=[]  KbParamMax=[]  KtParamMin=[]  KtParamMax=[]  POutMin=[]  POutMax=[]  IOutMin=[]  IOutMax=[]  DOutMin=[]  DOutMax=[]  NOutMin=[]  NOutMax=[]  KbOutMin=[]  KbOutMax=[]  KtOutMin=[]  KtOutMax=[]  IntegratorOutMin=[]  IntegratorOutMax=[]  FilterOutMin=[]  FilterOutMax=[]  SumOutMin=[]  SumOutMax=[]  SumI1OutMin=[]  SumI1OutMax=[]  SumI2OutMin=[]  SumI2OutMax=[]  SumI3OutMin=[]  SumI3OutMax=[]  SumDOutMin=[]  SumDOutMax=[]  SaturationOutMin=[]  SaturationOutMax=[]  IntegratorContinuousStateAttributes=''  IntegratorStateMustResolveToSignalObject=off  IntegratorRTWStateStorageClass=Auto  FilterContinuousStateAttributes=''  FilterStateMustResolveToSignalObject=off  FilterRTWStateStorageClass=Auto  DifferentiatorICPrevScaledInput=0  DifferentiatorOutMin=[]  DifferentiatorOutMax=[]
  Scale : Gain  Gain=RollMax
  Selector3 : Selector  InputPortWidth=3  IndexOptions=Index vector (dialog)  Indices=[1]  OutputSizes=1
  Sum : Sum  Inputs=|+-
  RollOut : Outport
  wires:
  Discrete PID Controller/1 -> RollOut/1
  Bus Selector/1 -> Selector3/1  "<RPY>"
  Selector3/1 -> Sum/2
  RollRef/1 -> Scale/1
  Bus/1 -> Bus Selector/1
  Scale/1 -> Sum/1
  Sum/1 -> Discrete PID Controller/1

== system A2Model/Controller/ManualCtrl/Mapper ==
  Thr : Inport
  Aileron : Inport  Port=2
  Elevator : Inport  Port=3
  Rudder : Inport  Port=4
  Bus Creator1 : BusCreator  Inputs=4
  Gain2 : Gain  Gain=-1
  LimitAndRescale : Subsystem
  LimitAndRescale1 : Subsystem
  LimitAndRescale2 : Subsystem
  LimitAndRescale3 : Subsystem
  PwmOut : Outport
  wires:
  LimitAndRescale3/1(ESCPWM) -> Bus Creator1/4  "PWM4"
  LimitAndRescale2/1(ESCPWM) -> Bus Creator1/3  "PWM3"
  Bus Creator1/1 -> PwmOut/1
  LimitAndRescale/1(ESCPWM) -> Bus Creator1/1  "PWM1"
  LimitAndRescale1/1(ESCPWM) -> Bus Creator1/2  "PWM2"
  Thr/1 -> LimitAndRescale/1(Scaled)
  Elevator/1 -> Gain2/1
  Aileron/1 -> LimitAndRescale1/1(Scaled)
  Gain2/1 -> LimitAndRescale2/1(Scaled)
  Rudder/1 -> LimitAndRescale3/1(Scaled)

== system A2Model/Controller/NextMode2/Mapper ==
  Thr : Inport
  Aileron : Inport  Port=2
  Elevator : Inport  Port=3
  Rudder : Inport  Port=4
  Bus Creator1 : BusCreator  Inputs=4
  Gain2 : Gain  Gain=-1
  LimitAndRescale : Subsystem
  LimitAndRescale1 : Subsystem
  LimitAndRescale2 : Subsystem
  LimitAndRescale3 : Subsystem
  PwmOut : Outport
  wires:
  LimitAndRescale3/1(ESCPWM) -> Bus Creator1/4  "PWM4"
  LimitAndRescale2/1(ESCPWM) -> Bus Creator1/3  "PWM3"
  Bus Creator1/1 -> PwmOut/1
  LimitAndRescale/1(ESCPWM) -> Bus Creator1/1  "PWM1"
  LimitAndRescale1/1(ESCPWM) -> Bus Creator1/2  "PWM2"
  Thr/1 -> LimitAndRescale/1(Scaled)
  Elevator/1 -> Gain2/1
  Aileron/1 -> LimitAndRescale1/1(Scaled)
  Gain2/1 -> LimitAndRescale2/1(Scaled)
  Rudder/1 -> LimitAndRescale3/1(Scaled)

== system A2Model/Controller/Off/Mapper ==
  Thr : Inport
  Aileron : Inport  Port=2
  Elevator : Inport  Port=3
  Rudder : Inport  Port=4
  Bus Creator1 : BusCreator  Inputs=4
  Gain2 : Gain  Gain=-1
  LimitAndRescale : Subsystem
  LimitAndRescale1 : Subsystem
  LimitAndRescale2 : Subsystem
  LimitAndRescale3 : Subsystem
  PwmOut : Outport
  wires:
  LimitAndRescale3/1(ESCPWM) -> Bus Creator1/4  "PWM4"
  LimitAndRescale2/1(ESCPWM) -> Bus Creator1/3  "PWM3"
  Bus Creator1/1 -> PwmOut/1
  LimitAndRescale/1(ESCPWM) -> Bus Creator1/1  "PWM1"
  LimitAndRescale1/1(ESCPWM) -> Bus Creator1/2  "PWM2"
  Thr/1 -> LimitAndRescale/1(Scaled)
  Elevator/1 -> Gain2/1
  Aileron/1 -> LimitAndRescale1/1(Scaled)
  Gain2/1 -> LimitAndRescale2/1(Scaled)
  Rudder/1 -> LimitAndRescale3/1(Scaled)

== system A2Model/Model/Environment/Gravity ==
  DCM : Inport
  Constant : Constant  Value=[0 0 -9.81]
  Mass : Gain  Gain=Mass
  Matrix Multiply : Product  Multiplication=Matrix(*)
  F[N] : Outport
  wires:
  Constant/1 -> Mass/1
  DCM/1 -> Matrix Multiply/1
  Matrix Multiply/1 -> F[N]/1
  Mass/1 -> Matrix Multiply/2

== system A2Model/Model/Propulsion/Servo ==
  note: Set to -1 for 1000
      | Set to 1 for 2000
  PWM : Inport
  AngleDEGOn1000 : Gain  Gain=90
  Constant1 : Constant  Value=1500  OutDataTypeStr=single
  Normalize : Gain  Gain=1/(2000-1500)
  Subtract1 : Sum  Inputs=+-
  Degree : Outport
  wires:
  Constant1/1 -> Subtract1/2
  Normalize/1 -> AngleDEGOn1000/1
  PWM/1 -> Subtract1/1
  Subtract1/1 -> Normalize/1
  AngleDEGOn1000/1 -> Degree/1

== system A2Model/Model/Propulsion/Servo1 ==
  note: Set to -1 for 1000
      | Set to 1 for 2000
  PWM : Inport
  AngleDEGOn1000 : Gain  Gain=90
  Constant1 : Constant  Value=1500  OutDataTypeStr=single
  Normalize : Gain  Gain=1/(2000-1500)
  Subtract1 : Sum  Inputs=+-
  Degree : Outport
  wires:
  Constant1/1 -> Subtract1/2
  Normalize/1 -> AngleDEGOn1000/1
  PWM/1 -> Subtract1/1
  Subtract1/1 -> Normalize/1
  AngleDEGOn1000/1 -> Degree/1

== system A2Model/Model/Propulsion/Servo2 ==
  note: Set to -1 for 1000
      | Set to 1 for 2000
  PWM : Inport
  AngleDEGOn1000 : Gain  Gain=90
  Constant1 : Constant  Value=1500  OutDataTypeStr=single
  Normalize : Gain  Gain=1/(2000-1500)
  Subtract1 : Sum  Inputs=+-
  Degree : Outport
  wires:
  Constant1/1 -> Subtract1/2
  Normalize/1 -> AngleDEGOn1000/1
  PWM/1 -> Subtract1/1
  Subtract1/1 -> Normalize/1
  AngleDEGOn1000/1 -> Degree/1

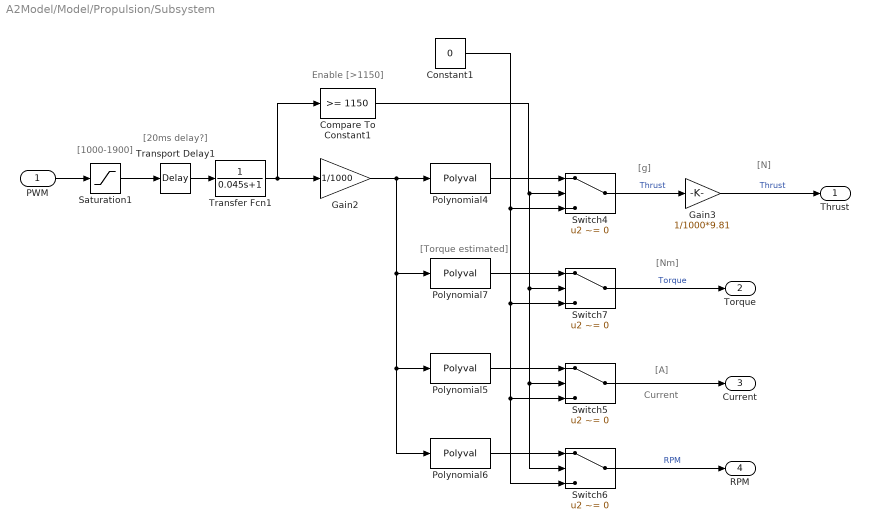
== system A2Model/Model/Propulsion/Subsystem ==
  note: [N]
  note: [g]
  note: [Nm]
  note: [A]
  note: [20ms delay?]
  note: [Torque estimated]
  note: [1000-1900]
  note: Current
  note: Enable [>1150]
  PWM : Inport  OutDataTypeStr=double  PortDimensions=1  SampleTime=0
  Compare To Constant1 : simulink/Logic and Bit Operations/Compare To Constant  relop=>=  const=1150  OutDataTypeStr=boolean
  Constant1 : Constant  Value=0
  Gain2 : Gain  Gain=1/1000
  Gain3 : Gain  Gain=1/1000*9.81
  Polynomial4 : Polyval  Coefs="[194.0242  232.6928 -846.8342  374.2523]"
  Polynomial5 : Polyval  Coefs="[23.1858  -80.9421   97.9875  -40.9978]"
  Polynomial6 : Polyval  Coefs="1.0e+04 *[-0.6016    2.6561   -2.8627    0.8887]"
  Polynomial7 : Polyval  Coefs="1e-3*0.11*[194.0242  232.6928 -846.8342  374.2523]"
  Saturation1 : Saturate  UpperLimit=1900  LowerLimit=1000
  Switch{4..7} (4 alike) : Switch  Criteria=u2 ~= 0
  Transfer Fcn1 : TransferFcn  Denominator=[0.045 1]
  Transport Delay1 : TransportDelay  DelayTime=0.02
  Thrust : Outport  OutDataTypeStr=double  PortDimensions=1  SampleTime=0
  Torque : Outport  Port=2  OutDataTypeStr=double  PortDimensions=1  SampleTime=0
  Current : Outport  Port=3  OutDataTypeStr=double  PortDimensions=1  SampleTime=0
  RPM : Outport  Port=4  OutDataTypeStr=double  PortDimensions=1  SampleTime=0
  wires:
  Gain3/1 -> Thrust/1  "Thrust"
  Saturation1/1 -> Transport Delay1/1
  Transport Delay1/1 -> Transfer Fcn1/1
  Gain2/1 -> Polynomial4/1, Polynomial6/1, Polynomial5/1, Polynomial7/1
  Compare To Constant1/1 -> Switch4/2, Switch6/2, Switch5/2, Switch7/2
  Polynomial4/1 -> Switch4/1
  Constant1/1 -> Switch4/3, Switch6/3, Switch5/3, Switch7/3
  Switch4/1 -> Gain3/1  "Thrust"
  Polynomial5/1 -> Switch5/1
  Switch5/1 -> Current/1
  Polynomial6/1 -> Switch6/1
  Switch6/1 -> RPM/1  "RPM"
  Polynomial7/1 -> Switch7/1
  Switch7/1 -> Torque/1  "Torque"
  Transfer Fcn1/1 -> Gain2/1, Compare To Constant1/1
  PWM/1 -> Saturation1/1

== system A2Model/Controller/AttitudeMode/Mapper/LimitAndRescale ==
  Scaled : Inport
  Constant : Constant  Value=1000  OutDataTypeStr=single
  Gain : Gain  Gain=(2000-1000)
  Limit3 : Saturate  UpperLimit=1  LowerLimit=0
  Subtract : Sum
  ESCPWM : Outport
  wires:
  Constant/1 -> Subtract/2
  Gain/1 -> Subtract/1
  Scaled/1 -> Limit3/1
  Subtract/1 -> ESCPWM/1
  Limit3/1 -> Gain/1

== system A2Model/Controller/AttitudeMode/Mapper/LimitAndRescale1 ==
  Scaled : Inport
  Constant : Constant  Value=1500  OutDataTypeStr=single
  Gain : Gain  Gain=(1500-1000)
  Limit3 : Saturate  UpperLimit=1  LowerLimit=-1
  Subtract : Sum
  ESCPWM : Outport
  wires:
  Constant/1 -> Subtract/2
  Gain/1 -> Subtract/1
  Scaled/1 -> Limit3/1
  Subtract/1 -> ESCPWM/1
  Limit3/1 -> Gain/1

== system A2Model/Controller/AttitudeMode/Mapper/LimitAndRescale2 ==
  Scaled : Inport
  Constant : Constant  Value=1500  OutDataTypeStr=single
  Gain : Gain  Gain=(1500-1000)
  Limit3 : Saturate  UpperLimit=1  LowerLimit=-1
  Subtract : Sum
  ESCPWM : Outport
  wires:
  Constant/1 -> Subtract/2
  Gain/1 -> Subtract/1
  Scaled/1 -> Limit3/1
  Subtract/1 -> ESCPWM/1
  Limit3/1 -> Gain/1

== system A2Model/Controller/AttitudeMode/Mapper/LimitAndRescale3 ==
  Scaled : Inport
  Constant : Constant  Value=1500  OutDataTypeStr=single
  Gain : Gain  Gain=(1500-1000)
  Limit3 : Saturate  UpperLimit=1  LowerLimit=-1
  Subtract : Sum
  ESCPWM : Outport
  wires:
  Constant/1 -> Subtract/2
  Gain/1 -> Subtract/1
  Scaled/1 -> Limit3/1
  Subtract/1 -> ESCPWM/1
  Limit3/1 -> Gain/1

== system A2Model/Controller/ManualCtrl/Mapper/LimitAndRescale ==
  Scaled : Inport
  Constant : Constant  Value=1000  OutDataTypeStr=single
  Gain : Gain  Gain=(2000-1000)
  Limit3 : Saturate  UpperLimit=1  LowerLimit=0
  Subtract : Sum
  ESCPWM : Outport
  wires:
  Constant/1 -> Subtract/2
  Gain/1 -> Subtract/1
  Scaled/1 -> Limit3/1
  Subtract/1 -> ESCPWM/1
  Limit3/1 -> Gain/1

== system A2Model/Controller/ManualCtrl/Mapper/LimitAndRescale1 ==
  Scaled : Inport
  Constant : Constant  Value=1500  OutDataTypeStr=single
  Gain : Gain  Gain=(1500-1000)
  Limit3 : Saturate  UpperLimit=1  LowerLimit=-1
  Subtract : Sum
  ESCPWM : Outport
  wires:
  Constant/1 -> Subtract/2
  Gain/1 -> Subtract/1
  Scaled/1 -> Limit3/1
  Subtract/1 -> ESCPWM/1
  Limit3/1 -> Gain/1

== system A2Model/Controller/ManualCtrl/Mapper/LimitAndRescale2 ==
  Scaled : Inport
  Constant : Constant  Value=1500  OutDataTypeStr=single
  Gain : Gain  Gain=(1500-1000)
  Limit3 : Saturate  UpperLimit=1  LowerLimit=-1
  Subtract : Sum
  ESCPWM : Outport
  wires:
  Constant/1 -> Subtract/2
  Gain/1 -> Subtract/1
  Scaled/1 -> Limit3/1
  Subtract/1 -> ESCPWM/1
  Limit3/1 -> Gain/1

== system A2Model/Controller/ManualCtrl/Mapper/LimitAndRescale3 ==
  Scaled : Inport
  Constant : Constant  Value=1500  OutDataTypeStr=single
  Gain : Gain  Gain=(1500-1000)
  Limit3 : Saturate  UpperLimit=1  LowerLimit=-1
  Subtract : Sum
  ESCPWM : Outport
  wires:
  Constant/1 -> Subtract/2
  Gain/1 -> Subtract/1
  Scaled/1 -> Limit3/1
  Subtract/1 -> ESCPWM/1
  Limit3/1 -> Gain/1

== system A2Model/Controller/NextMode2/Mapper/LimitAndRescale ==
  Scaled : Inport
  Constant : Constant  Value=1000  OutDataTypeStr=single
  Gain : Gain  Gain=(2000-1000)
  Limit3 : Saturate  UpperLimit=1  LowerLimit=0
  Subtract : Sum
  ESCPWM : Outport
  wires:
  Constant/1 -> Subtract/2
  Gain/1 -> Subtract/1
  Scaled/1 -> Limit3/1
  Subtract/1 -> ESCPWM/1
  Limit3/1 -> Gain/1

== system A2Model/Controller/NextMode2/Mapper/LimitAndRescale1 ==
  Scaled : Inport
  Constant : Constant  Value=1500  OutDataTypeStr=single
  Gain : Gain  Gain=(1500-1000)
  Limit3 : Saturate  UpperLimit=1  LowerLimit=-1
  Subtract : Sum
  ESCPWM : Outport
  wires:
  Constant/1 -> Subtract/2
  Gain/1 -> Subtract/1
  Scaled/1 -> Limit3/1
  Subtract/1 -> ESCPWM/1
  Limit3/1 -> Gain/1

== system A2Model/Controller/NextMode2/Mapper/LimitAndRescale2 ==
  Scaled : Inport
  Constant : Constant  Value=1500  OutDataTypeStr=single
  Gain : Gain  Gain=(1500-1000)
  Limit3 : Saturate  UpperLimit=1  LowerLimit=-1
  Subtract : Sum
  ESCPWM : Outport
  wires:
  Constant/1 -> Subtract/2
  Gain/1 -> Subtract/1
  Scaled/1 -> Limit3/1
  Subtract/1 -> ESCPWM/1
  Limit3/1 -> Gain/1

== system A2Model/Controller/NextMode2/Mapper/LimitAndRescale3 ==
  Scaled : Inport
  Constant : Constant  Value=1500  OutDataTypeStr=single
  Gain : Gain  Gain=(1500-1000)
  Limit3 : Saturate  UpperLimit=1  LowerLimit=-1
  Subtract : Sum
  ESCPWM : Outport
  wires:
  Constant/1 -> Subtract/2
  Gain/1 -> Subtract/1
  Scaled/1 -> Limit3/1
  Subtract/1 -> ESCPWM/1
  Limit3/1 -> Gain/1

== system A2Model/Controller/Off/Mapper/LimitAndRescale ==
  Scaled : Inport
  Constant : Constant  Value=1000  OutDataTypeStr=single
  Gain : Gain  Gain=(2000-1000)
  Limit3 : Saturate  UpperLimit=1  LowerLimit=0
  Subtract : Sum
  ESCPWM : Outport
  wires:
  Constant/1 -> Subtract/2
  Gain/1 -> Subtract/1
  Scaled/1 -> Limit3/1
  Subtract/1 -> ESCPWM/1
  Limit3/1 -> Gain/1

== system A2Model/Controller/Off/Mapper/LimitAndRescale1 ==
  Scaled : Inport
  Constant : Constant  Value=1500  OutDataTypeStr=single
  Gain : Gain  Gain=(1500-1000)
  Limit3 : Saturate  UpperLimit=1  LowerLimit=-1
  Subtract : Sum
  ESCPWM : Outport
  wires:
  Constant/1 -> Subtract/2
  Gain/1 -> Subtract/1
  Scaled/1 -> Limit3/1
  Subtract/1 -> ESCPWM/1
  Limit3/1 -> Gain/1

== system A2Model/Controller/Off/Mapper/LimitAndRescale2 ==
  Scaled : Inport
  Constant : Constant  Value=1500  OutDataTypeStr=single
  Gain : Gain  Gain=(1500-1000)
  Limit3 : Saturate  UpperLimit=1  LowerLimit=-1
  Subtract : Sum
  ESCPWM : Outport
  wires:
  Constant/1 -> Subtract/2
  Gain/1 -> Subtract/1
  Scaled/1 -> Limit3/1
  Subtract/1 -> ESCPWM/1
  Limit3/1 -> Gain/1

== system A2Model/Controller/Off/Mapper/LimitAndRescale3 ==
  Scaled : Inport
  Constant : Constant  Value=1500  OutDataTypeStr=single
  Gain : Gain  Gain=(1500-1000)
  Limit3 : Saturate  UpperLimit=1  LowerLimit=-1
  Subtract : Sum
  ESCPWM : Outport
  wires:
  Constant/1 -> Subtract/2
  Gain/1 -> Subtract/1
  Scaled/1 -> Limit3/1
  Subtract/1 -> ESCPWM/1
  Limit3/1 -> Gain/1

== stateflow chart A2Model/Controller/Chart ==
  state SystemLogic [parallel]
    en: Mode = uint8(0);
    du: SelectMode()
    settings: executionOrder=2
    state ActiveModes
      en:
      ModeOld = Mode;
      state ManualMode
        entry:
        ActualMode=uint8(1);
      state AttitudeMode
        entry:
        ActualMode=uint8(2);
      state ArcadeMode
        entry:
        ActualMode=uint8(3);
    state Off
      entry:
      ActualMode=uint8(0);
    state SelectMode [function]
      (default) -> (junction 20)
      (junction 20) -> (junction 21) [order 1] : [ ModeInput < 600 ]
      (junction 21) -> (junction 22) : {Mode = uint8(1);}
      (junction 22) -> (junction 25)
      (junction 20) -> (junction 23) [order 2]
      (junction 23) -> (junction 24) [order 1] : [ ModeInput < 1300 ]
      (junction 24) -> (junction 25) : {Mode = uint8(2);}
      (junction 23) -> (junction 26) [order 2] : {Mode = uint8(3);}
      (junction 25) -> (junction 27)
      (junction 27) -> (junction 26)
      (junction 26) -> (junction 28)
    (default) -> Off
    Off -> ManualMode [order 1] : [Mode==1]
    Off -> AttitudeMode [order 2] : [Mode==2]
    Off -> ArcadeMode [order 3] : [Mode==3]
    ActiveModes -> Off : [ Mode ~= ModeOld ]
  state LEDs [parallel]
    settings: executionOrder=1
    state GreenOn
      entry: LED = true;
    state GreenOff
      entry: LED = false;
    (default) -> GreenOn
    GreenOn -> GreenOff : [after(100,tick)]
    GreenOff -> GreenOn : [after(100,tick)]
  data: LED output boolean size=1; ActualMode output uint8; Off output boolean; Mode local uint8; ModeOld local uint8; ManualMode output boolean; AttitudeMode output boolean; ArcadeMode output boolean; ModeInput input uint32

== matlab function A2Model/Controller/AltCalculator/MATLAB Function ==
  data: pressure input; alt output; pressure0 input
function alt = fcn(pressure, pressure0)
%#codegen
if (pressure < 10000) || (pressure > 150000) % pressure not valid?
    alt = single(0);
else
    alt = 44330*(1-(pressure/pressure0)^(1/5.255));    
end
